simulink model "cop"  (R2024a)
settings: Solver=VariableStepAuto  StartTime=0.0  StopTime=2000  RelTol=1e-3
undefined symbols (not defined in the file): b, g, JB, k, L_COM, mB
libraries: slpidlib x1
settings Model: Creator=lenovo  LastModifiedBy=lenovo

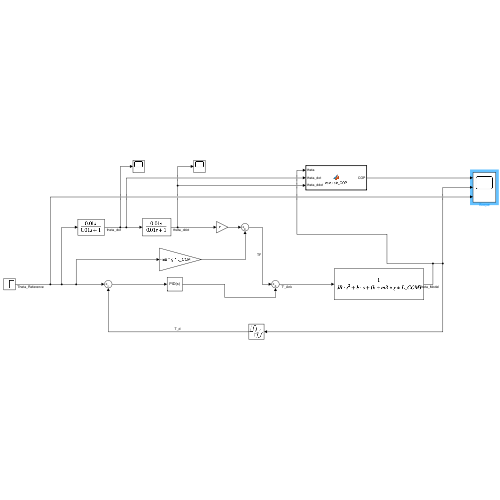
[thumbnail: Simulink's stored preview of the top-level diagram]
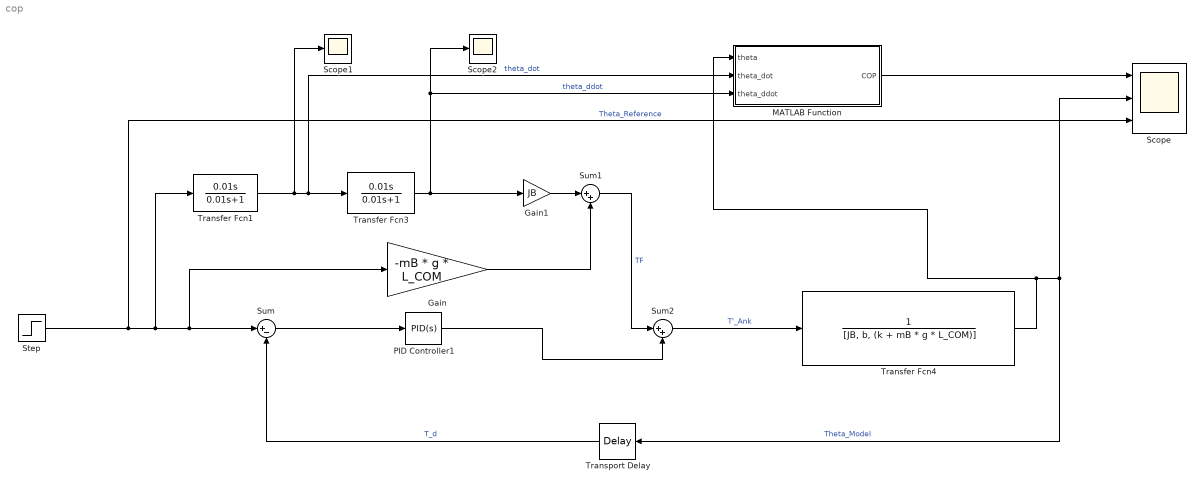
== system cop ==
  Gain : Gain  Gain=-mB * g * L_COM
  Gain1 : Gain  Gain=JB
  MATLAB Function : MATLAB Function  TreatAsAtomicUnit=on
  PID Controller1 : slpidlib/PID Controller  Controller=PID  Form=Parallel  TimeDomain=Continuous-time  UseExternalTs=off  SampleTime=-1  IntegratorMethod=Forward Euler  FilterMethod=Forward Euler  ControllerParametersSource=internal  P=3.69  I=3.36986301  UseKiTs=off  D=250  UseExternalDerivativeSource=off  N=100  UseFilter=on  TunerSelectOption=Transfer Function Based (PID Tuner App)  InitialConditionSource=internal  InitialConditionForIntegrator=0  InitialConditionForFilter=0  DifferentiatorICPrevScaledInput=0  ExternalReset=none  TrackingMode=off  Kt=1  LimitOutput=off  SatLimitsSource=internal  UpperSaturationLimit=inf  LowerSaturationLimit=-inf  LinearizeAsGain=on  AntiWindupMode=none  Kb=1  LimitIntegrator=off  UpperIntegratorSaturationLimit=inf  LowerIntegratorSaturationLimit=-inf  POutMin=[]  POutMax=[]  IOutMin=[]  IOutMax=[]  DOutMin=[]  DOutMax=[]  NOutMin=[]  NOutMax=[]  SumOutMin=[]  SumOutMax=[]  SaturationOutMin=[]  SaturationOutMax=[]  PParamMin=[]  PParamMax=[]  IParamMin=[]  IParamMax=[]  DParamMin=[]  DParamMax=[]  NParamMin=[]  NParamMax=[]  KbParamMin=[]  KbParamMax=[]  KtParamMin=[]  KtParamMax=[]  KbOutMin=[]  KbOutMax=[]  KtOutMin=[]  KtOutMax=[]  IntegratorOutMin=[]  IntegratorOutMax=[]  FilterOutMin=[]  FilterOutMax=[]  SumI1OutMin=[]  SumI1OutMax=[]  SumI2OutMin=[]  SumI2OutMax=[]  SumI3OutMin=[]  SumI3OutMax=[]  SumI4OutMin=[]  SumI4OutMax=[]  SumDOutMin=[]  SumDOutMax=[]  DifferentiatorOutMin=[]  DifferentiatorOutMax=[]  FilterDiffOutCoefMin=[]  FilterDiffOutCoefMax=[]  ReciprocalOutMin=[]  ReciprocalOutMax=[]  SumDenOutMin=[]  SumDenOutMax=[]  SumNumOutMin=[]  SumNumOutMax=[]  DivideOutMin=[]  DivideOutMax=[]  UdiffTsProdOutMin=[]  UdiffTsProdOutMax=[]  NTsProdOutMin=[]  NTsProdOutMax=[]  UintegralTsProdOutMin=[]  UintegralTsProdOutMax=[]  UngainTsProdOutMin=[]  UngainTsProdOutMax=[]  ClampingZeroOutDataTypeStr=Inherit: Inherit via back propagation  ClampingZeroOutMin=[]  ClampingZeroOutMax=[]  FilterDenConstantOutDataTypeStr=Inherit: Inherit via back propagation  FilterDenConstantOutMin=[]  FilterDenConstantOutMax=[]  PCopyOutDataTypeStr=Inherit: Inherit via back propagation  PCopyOutMin=[]  PCopyOutMax=[]  NCopyOutDataTypeStr=Inherit: Inherit via back propagation  NCopyOutMin=[]  NCopyOutMax=[]  IntegratorContinuousStateAttributes=''  IntegratorStateMustResolveToSignalObject=off  IntegratorRTWStateStorageClass=Auto  FilterContinuousStateAttributes=''  FilterStateMustResolveToSignalObject=off  FilterRTWStateStorageClass=Auto  ParallelPVariant=InternalParameters  IdealPVariant=Disabled  IVariant=InternalParameters  DVariant=InternalParameters  IntegratorVariant=Continuous  SatVariant=Disabled  AWVariant=Passthrough  PCopyVariant=Disabled  TRVariant=Disabled  FdbkBlocksVariant=Forward  IdealPFdbkVariant=Disabled  SatFdbkVariant=Disabled  DerivativeFilterVariant=ContFilter  NVariant=InternalParameters  NCopyVariant=Disabled  FilterICVariant=InternalICsFilter  IntegratorICVariant=InternalICs  ExternalResetVariant=Disabled  TRSumVariant=Passthrough  SumFdbkVariant=Disabled  SumVariant=Sum_PID  TsampFilterVariant=InternalTs  TsampNgainVariant=Passthrough  TsampIntegralVariant=Disabled_SignalSpec  ExternalSaturationOutDataTypeStr=Inherit: Same as second input  DerivativeSourceVariant=ErrorSignal
  Scope : Scope  NumInputPorts=3
  Scope1 : Scope
  Scope2 : Scope
  Step : Step  SampleTime=0
  Sum : Sum  Inputs=|+-
  Sum1 : Sum  Inputs=|++
  Sum2 : Sum  Inputs=|++
  Transfer Fcn1 : TransferFcn  Numerator=[0.01, 0]  Denominator=[0.01, 1]
  Transfer Fcn3 : TransferFcn  Numerator=[0.01, 0]  Denominator=[0.01, 1]
  Transfer Fcn4 : TransferFcn  Denominator=[JB, b, (k + mB * g * L_COM)]
  Transport Delay : TransportDelay  DelayTime=0.171
  wires:
  Gain/1 -> Sum1/2
  Transfer Fcn1/1 -> MATLAB Function/2(theta_dot), Transfer Fcn3/1, Scope1/1  "theta_dot"
  Transfer Fcn3/1 -> Gain1/1, Scope2/1, MATLAB Function/3(theta_ddot)  "theta_ddot"
  Gain1/1 -> Sum1/1
  Sum1/1 -> Sum2/1  "TF"
  Sum/1 -> PID Controller1/1
  Transport Delay/1 -> Sum/2  "T_d"
  Sum2/1 -> Transfer Fcn4/1  "T'_Ank"
  Step/1 -> Scope/3, Transfer Fcn1/1, Sum/1, Gain/1  "Theta_Reference"
  Transfer Fcn4/1 -> MATLAB Function/1(theta), Transport Delay/1, Scope/2  "Theta_Model"
  MATLAB Function/1(COP) -> Scope/1
  PID Controller1/1 -> Sum2/2

== matlab function cop/MATLAB Function ==
  data: theta input; COP output; theta_dot input; theta_ddot input
function COP = calculate_COP(theta, theta_dot, theta_ddot)
% Calculate the Center of Pressure (COP) based on the body lean angle and its derivatives

% Define constants (or pass them as inputs)
mB = 70;          % Mass of the body (kg)
mF = 2;           % Mass of the feet (kg)
g = 9.81;         % Acceleration due to gravity (m/s^2)
L_COM = 0.9;      % Distance from ankle to body's center of mass (m)
JB = (1/3) * mB * (1.8)^2;  % Moment of inertia (kg·m^2)
xF = 0;           % Horizontal position of foot COM (m)
zF = 0;           % Height of ankle joint (m)

% Calculate vertical acceleration of the body's center of mass (aBz)
aBz = -L_COM * theta_ddot * cos(theta) + L_COM * theta_dot^2 * sin(theta);

% Numerator of COP equation
numerator = -JB * theta_ddot + mB * g * L_COM * theta + mF * g * xF - mB * aBz * zF;

% Denominator of COP equation
denominator = mB * aBz + mB * g + mF * g;

% Prevent division by zero
epsilon = 1e-6;
if abs(denominator) < epsilon
    denominator = epsilon;
end

% Calculate COP
COP = numerator / denominator;
end
